simulink model "warplab_mimo_4x4"  (Simulink 6.6)
settings: Solver=ode45  StartTime=0.0  StopTime=50000  RelTol=1e-3
undefined symbols (not defined in the file): gcbh, xlBlockLoadCallback, xlGetSimulinkPeriod
libraries: xbsIndex_r4 x305, WARP_Blockset x16
(part 1 of 4)
settings Model: Creator=mduarte  LastModifiedBy=mduarte

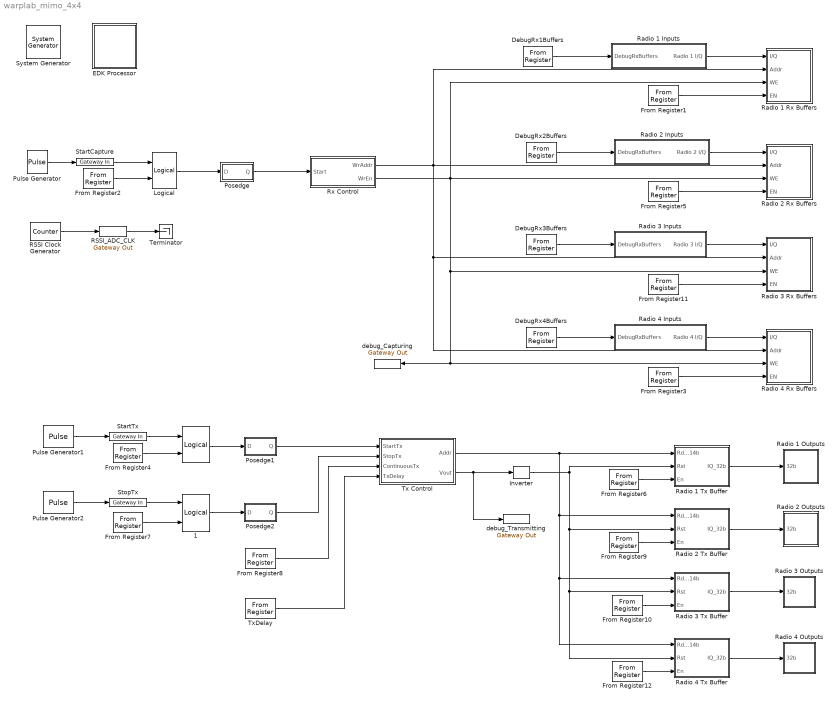
== system warplab_mimo_4x4 ==
  " " : xbsIndex_r4/Logical  logical_function=OR  inputs=2  en=off  latency=0  precision=Full  arith_type=Unsigned  n_bits=16  bin_pt=0  align_bp=on  dbl_ovrd=off  block_type=logical
      settings: block_version=9.1.01
  " 1" : xbsIndex_r4/Logical  logical_function=OR  inputs=2  en=off  latency=0  precision=Full  arith_type=Unsigned  n_bits=16  bin_pt=0  align_bp=on  dbl_ovrd=off  block_type=logical
      settings: block_version=9.1.01
  " System Generator" : xbsIndex_r4/ System Generator  Tag=genX  SystemSampleTime=-1  xilinxfamily=virtex2p  part=xc2vp70  speed=-6  package=ff1517  synthesis_tool=XST  clock_wrapper=Clock Enables  directory=./netlist  testbench=off  simulink_period=1  sysclk_period=10  dcm_input_clock_period=100  incr_netlist=off  trim_vbits=Everywhere in SubSystem  dbl_ovrd=According to Block Masks  core_generation=According to Block Masks  run_coregen=off  deprecated_control=off  eval_field=0  block_type=sysgen
      settings: block_version=10.1.3
  DebugRx1Buffers : xbsIndex_r4/From Register  shared_memory_name='DebugRx1Buffers'  init=0  period=1  ownership=Locally owned and initialized  arith_type=Unsigned  n_bits=1  bin_pt=0  dbl_ovrd=off  block_type=fromreg
      settings: AttributesFormatString=<< %<shared_memory_name> >>  infoedit="Register block that reads data to a shared memory register.  Delay of one sample period."  block_version=10.1.2
  DebugRx2Buffers : xbsIndex_r4/From Register  shared_memory_name='DebugRx2Buffers'  init=0  period=1  ownership=Locally owned and initialized  arith_type=Unsigned  n_bits=1  bin_pt=0  dbl_ovrd=off  block_type=fromreg
      settings: AttributesFormatString=<< %<shared_memory_name> >>  infoedit="Register block that reads data to a shared memory register.  Delay of one sample period."  block_version=10.1.2
  DebugRx3Buffers : xbsIndex_r4/From Register  shared_memory_name='DebugRx3Buffers'  init=0  period=1  ownership=Locally owned and initialized  arith_type=Unsigned  n_bits=1  bin_pt=0  dbl_ovrd=off  block_type=fromreg
      settings: AttributesFormatString=<< %<shared_memory_name> >>  infoedit="Register block that reads data to a shared memory register.  Delay of one sample period."  block_version=10.1.2
  DebugRx4Buffers : xbsIndex_r4/From Register  shared_memory_name='DebugRx4Buffers'  init=0  period=1  ownership=Locally owned and initialized  arith_type=Unsigned  n_bits=1  bin_pt=0  dbl_ovrd=off  block_type=fromreg
      settings: AttributesFormatString=<< %<shared_memory_name> >>  infoedit="Register block that reads data to a shared memory register.  Delay of one sample period."  block_version=10.1.2
  EDK Processor : Subsystem  LoadFcn=xlBlockLoadCallback(gcbh);  mask(Xilinx EDK Processor Block){mode=EDK pcore generation, xmp=, MemVisToProc=<qt bgcolor="#FFFFFF"><div><img src="C:\Xilinx\10.1\DSP_Tools\sysgen\data\images\registerplus.gif"> &lt;&lt;CaptureDone&gt;&gt;<br></div><div><img src="C:\Xilinx\10.1\DSP_Tools\sysgen\data\images\registerplus.gif"> &lt;&lt;DebugRx1Buffers&gt;&gt;<br></div><div><img src="C:\Xilinx\10.1\DSP_Tools\sysgen\data\images\registerplus.gif"> &lt;&lt;DebugRx2Buffers&gt;&gt;<br></div><div><img src="C:\Xilinx\10.1\DSP_Tools\sysgen\data\images\registerplus.gif"> &lt;&lt;DebugRx3Buffers&gt;&gt;<br></div><div><img src="C:\Xilinx\10.1\DSP_Tools\sysgen\data\images\registerplus.gif"> &lt;&lt;DebugRx4Buffers&gt;&gt;<br></div><div><img src="C:\Xilinx\10.1\DSP_Tools\sysgen\data\images\registerplus.gif"> &lt;&lt;RADIO1RXBUFF_RXEN&gt;&gt;<br></div><div><img src="C:\Xilinx\10.1\DSP_Tools\sysgen\data\images\registerplus.gif"> &lt;&lt;RADIO1TXBUFF_TXEN&gt;&gt;<br></div><div><img src="C:\Xilinx\10.1\DSP_Tools\sysgen\data\images\registerplus.gif"> &lt;&lt;RADIO2RXBUFF_RXEN&gt;&gt;<br></div><div><img src="C:\Xilinx\10.1\DSP_Tools\sysgen\data\images\registerplus.gif"> &lt;&lt;RADIO2TXBUFF_TXEN&gt;&gt;<br></div><div><img src="C:\Xilinx\10.1\DSP_Tools\sysgen\data\images\registerplus.gif"> &lt;&lt;RADIO3RXBUFF_RXEN&gt;&gt;<br></div><div><img src="C:\Xilinx\10.1\DSP_Tools\sysgen\data\images\registerplus.gif"> &lt;&lt;RADIO3TXBUFF_TXEN&gt;&gt;<br></div><div><img src="C:\Xilinx\10.1\DSP_Tools\sysgen\data\images\registerplus.gif"> &lt;&lt;RADIO4RXBUFF_RXEN&gt;&gt;<br></div><div><img src="C:\Xilinx\10.1\DSP_Tools\sysgen\data\images\registerplus.gif"> &lt;&lt;RADIO4TXBUFF_TXEN&gt;&gt;<br></div><div><img src="C:\Xilinx\10.1\DSP_Tools\sysgen\data\images\registerplus.gif"> &lt;&lt;StartCapture&gt;&gt;<br></div><div><img src="C:\Xilinx\10.1\DSP_Tools\sysgen\data\images\registerplus.gif"> &lt;&lt;StartTx&gt;&gt;<br></div><div><img src="C:\Xilinx\10.1\DSP_Tools\sysgen\data\images\registerplus.gif"> &lt;&lt;StopTx&gt;&gt;<br></div><div><img src="C:\Xilinx\10.1\DSP_Tools\sysgen\data\images\registerplus.gif"> &lt;&lt;TransMode&gt;&gt;<br></div><div><img src="C:\Xilinx\10.1\DSP_Tools\sysgen\data\images\registerplus.gif"> &lt;&lt;TxDelay&gt;&gt;<br></div><div><img src="C:\Xilinx\10.1\DSP_Tools\sysgen\data\images\registerplus.gif"> &lt;&lt;TxLength&gt;&gt;<br></div><div><img src="C:\Xilinx\10.1\DSP_Tools\sysgen\data\images\memoryplus.gif"> &lt;&lt;RxBuff_Radio1&gt;&gt;<br></div><div><img src="C:\Xilinx\10.1\DSP_Tools\sysgen\data\images\memoryplus.gif"> &lt;&lt;RxBuff_Radio2&gt;&gt;<br></div><div><img src="C:\Xilinx\10.1\DSP_Tools\sysgen\data\images\memoryplus.gif"> &lt;&lt;RxBuff_Radio3&gt;&gt;<br></div><div><img src="C:\Xilinx\10.1\DSP_Tools\sysgen\data\images\memoryplus.gif"> &lt;&lt;RxBuff_Radio4&gt;&gt;<br></div><div><img src="C:\Xilinx\10.1\DSP_Tools\sysgen\data\images\memoryplus.gif"> &lt;&lt;TxBuff_Radio1&gt;&gt;<br></div><div><img src="C:\Xilinx\10.1\DSP_Tools\sysgen\data\images\memoryplus.gif"> &lt;&lt;TxBuff_Radio2&gt;&gt;<br></div><div><img src="C:\Xilinx\10.1\DSP_Tools\sysgen\data\images\memoryplus.gif"> &lt;&lt;TxBuff_Radio3&gt;&gt;<br></div><div><img src="C:\Xilinx\10.1\DSP_Tools\sysgen\data\images\memoryplus.gif"> &lt;&lt;TxBuff_Radio4&gt;&gt;<br></div></qt>, AvailableMemories=<empty>, portInterfaceTable={'exposed'=>[],'portdir'=>[],'portname'=>[],'shortname'=>[]}, bus_type_sgadvanced=, bus_type=PLB, baseaddr=0x80000000, baseaddr_lock_sgadvanced=, baseaddr_lock=off, dual_clock_sgadvanced=, dual_clock=on, reg_readback_sgadvanced=, reg_readback=on, ucf_file=, inheritDeviceType_sgadvanced=, inheritDeviceType=off, clock_name=plb, internalPortList={}, resetPolarity=0, memxtable=|, procinfo={'xmliface'=>'Xilinx//microblaze//iface.xml'}, memmapdirty=off, blockname=, xpsintstyle=default, has_advanced_control=0, sggui_pos=20,20,383,441, block_type=edkprocessor, block_version=2.5, sg_icon_stat=62,64,-1,-1,white,blue,0,07734,right, sg_mask_display=|, sg_list_contents={'table'=>{'AvailableMemories'=>'popup(<empty>)','userSelections'=>{'AvailableMemories'=>'<empty>'}}}, sg_blockgui_xml=}
      mask memxtable=|
      | {'mlist'=>['warplab_mimo_4x4/Rx Control/To Register','warplab_mimo_4x4/DebugRx1Buffers','warplab_mimo_4x4/DebugRx2Buffers','warplab_mimo_4x4/DebugRx3Buffers','warplab_mimo_4x4/DebugRx4Buffers','warplab_mimo_4x4/From Register1','warplab_mimo_4x4/From Register6','warplab_mimo_4x4/From Register5','warplab_mimo_4x4/From Register9','warplab_mimo_4x4/From Register11','warplab_mimo_4x4/From Register10','warplab_mimo_4x4/From Register3','warplab_mimo_4x4/From Register12','warplab_mimo_4x4/From Register2','warplab_mimo_4x4/From Register4','warplab_mimo_4x4/From Register7','warplab_mimo_4x4/From Register8','warplab_mimo_4x4/TxDelay','warplab_mimo_4x4/Tx Control/From Register4','warplab_mimo_4x4/Radio 1
      | Rx Buffers/Radio 1 I//Q
      | Buffer/Shared Memory','warplab_mimo_4x4/Radio 2
      | Rx Buffers/Radio 2 I//Q
      | Buffer/Shared Memory','warplab_mimo_4x4/Radio 3
      | Rx Buffers/Radio 3 I//Q
      | Buffer/Shared Memory','warplab_mimo_4x4/Radio 4
      | Rx Buffers/Radio 4 I//Q
      | Buffer/Shared Memory','warplab_mimo_4x4/Radio 1
      | Tx Buffer/Shared Memory','warplab_mimo_4x4/Radio 2
      | Tx Buffer/Shared Memory','warplab_mimo_4x4/Radio 3
      | Tx Buffer/Shared Memory','warplab_mimo_4x4/Radio 4
      | Tx Buffer/Shared Memory'],'mlname'=>['\'CaptureDone\'','\'DebugRx1Buffers\'','\'DebugRx2Buffers\'','\'DebugRx3Buffers\'','\'DebugRx4Buffers\'','\'RADIO1RXBUFF_RXEN\'','\'RADIO1TXBUFF_TXEN\'','\'RADIO2RXBUFF_RXEN\'','\'RADIO2TXBUFF_TXEN\'','\'RADIO3RXBUFF_RXEN\'','\'RADIO3TXBUFF_TXEN\'','\'RADIO4RXBUFF_RXEN\'','\'RADIO4TXBUFF_TXEN\'','\'StartCapture\'','\'StartTx\'','\'StopTx\'','\'TransMode\'','\'TxDelay\'','\'TxLength\'','\'RxBuff_Radio1\'','\'RxBuff_Radio2\'','\'RxBuff_Radio3\'','\'RxBuff_Radio4\'','\'TxBuff_Radio1\'','\'TxBuff_Radio2\'','\'TxBuff_Radio3\'','\'TxBuff_Radio4\''],'mlstate'=>[0.00000000000000000,0.00000000000000000,0.00000000000000000,0.00000000000000000,0.00000000000000000,0.00000000000000000,0.00000000000000000,0.00000000000000000,0.00000000000000000,0.00000000000000000,0.00000000000000000,0.00000000000000000,0.00000000000000000,0.00000000000000000,0.00000000000000000,0.00000000000000000,0.00000000000000000,0.00000000000000000,0.00000000000000000,0.00000000000000000,0.00000000000000000,0.00000000000000000,0.00000000000000000,0.00000000000000000,0.00000000000000000,0.00000000000000000,0.00000000000000000]}
      mask sg_mask_display=|
      | fprintf('','COMMENT: begin icon graphics');
      | patch([0 62 62 0 ],[0 0 64 64 ],[0.77 0.82 0.91]);
      | patch([14 4 19 4 14 30 34 38 56 42 29 19 33 19 29 42 56 38 34 30 14 ],[8 18 33 48 58 58 54 58 58 44 57 47 33 19 9 22 8 8 12 8 8 ],[0.98 0.96 0.92]);
      | plot([0 62 62 0 0 ],[0 0 64 64 0 ]);
      | fprintf('','COMMENT: end icon graphics');
      | fprintf('','COMMENT: begin icon text');
      | fprintf('','COMMENT: end icon text');
      mask prompts: mode "Configure Processor for"; xmp "EDK Project"; MemVisToProc ""; AvailableMemories "Available Memories"; portInterfaceTable ""; bus_type_sgadvanced ""; bus_type "Bus Type"; baseaddr "Base Address"; baseaddr_lock_sgadvanced ""; baseaddr_lock "Lock"; dual_clock_sgadvanced ""; dual_clock "Dual Clocks"; reg_readback_sgadvanced ""; reg_readback "Register Read-Back"; ucf_file "Constraint file"; inheritDeviceType_sgadvanced ""; inheritDeviceType "Inherit Device Type"; clock_name ""; internalPortList ""; resetPolarity ""; memxtable ""; procinfo ""; memmapdirty ""; blockname ""; xpsintstyle ""; has_advanced_control ""; sggui_pos ""; block_type ""; block_version ""; sg_icon_stat ""; sg_mask_display ""; sg_list_contents ""; sg_blockgui_xml ""
      mask help: Xilinx EDK Processor
      mask init:
      | try
      |   tmp_gcb = gcb;
      |   tmp_gcbh = gcbh;
      |   if (strcmp('SysGenIndex',get_param(bdroot(tmp_gcbh),'tag')) && ~isempty(regexp(bdroot(tmp_gcb), '^xbs', 'once')))
      |     return;
      |   end;
      |   xlMungeMaskParams;
      | 
      | block_type='edkprocessor';
      |   serialized_declarations = '{,''block_type''=>''String''}';
      |   xledkprocessor_init();
      |   ptable_ = xlblockprep(get_param(tmp_gcb, 'MaskWSVariables'));
      | catch
      |   global dbgsysgen;
      |   if(~isempty(dbgsysgen) && dbgsysgen)
      |     e = regexprep(lasterr, '\n', '\nError: ');
      |     disp(['Error: While running MaskInit code on block ' tmp_gcb ': ' e]);
      |     error(e);
      |   end
      | end
      settings: CopyFcn=xlProcBlockCopyCallback(gcbh);xlBlockMoveCallback(gcbh);  DeleteFcn=xlDestroyGui(gcbh);  ModelCloseFcn=xlDestroyGui(gcbh);  PreSaveFcn=xlBlockPreSaveCallback(gcbh);  PostSaveFcn=xlBlockPostSaveCallback(gcbh);  DestroyFcn=xlDestroyGui(gcbh);  OpenFcn=bh=gcbh;xlProcBlockCallbacks('populatesharedmemorylistbox',bh);xlOpenGui(bh, 'edkprocessor_gui.xml', @xlProcBlockEnablement, @xlProcBlockAction)  CloseFcn=xlDestroyGui(gcbh);  MoveFcn=xlBlockMoveCallback(gcbh);
      mask Help: eval('');xlDoc('-book','sysgen','-topic','EDK_Processor');
      mask StyleString: popup(EDK pcore generation|HDL netlisting),edit,edit,popup(<empty>),edit,edit,popup(PLB|FSL),edit,edit,checkbox,edit,checkbox,edit,checkbox,edit,edit,checkbox,edit,edit,edit,edit,edit,edit,edit,edit,edit,edit,edit,edit,edit,edit,edit,edit
      mask Display:
      | fprintf('','COMMENT: begin icon graphics');
      | patch([0 62 62 0 ],[0 0 64 64 ],[0.77 0.82 0.91]);
      | patch([14 4 19 4 14 30 34 38 56 42 29 19 33 19 29 42 56 38 34 30 14 ],[8 18 33 48 58 58 54 58 58 44 57 47 33 19 9 22 8 8 12 8 8 ],[0.98 0.96 0.92]);
      | plot([0 62 62 0 0 ],[0 0 64 64 0 ]);
      | fprintf('','COMMENT: end icon graphics');
      | fprintf('','COMMENT: begin icon text');
      | disp('');
      | 
      | fprintf('','COMMENT: end icon text');
  From Register1 : xbsIndex_r4/From Register  shared_memory_name='RADIO1RXBUFF_RXEN'  init=0  period=1  ownership=Locally owned and initialized  arith_type=Unsigned  n_bits=1  bin_pt=0  dbl_ovrd=off  block_type=fromreg
      settings: AttributesFormatString=RADIO1RXBUFF_RXEN\n<< %<shared_memory_name> >>  infoedit="Register block that reads data to a shared memory register.  Delay of one sample period."  block_version=8.2
  From Register10 : xbsIndex_r4/From Register  shared_memory_name='RADIO3TXBUFF_TXEN'  init=0  period=1  ownership=Locally owned and initialized  arith_type=Unsigned  n_bits=1  bin_pt=0  dbl_ovrd=off  block_type=fromreg
      settings: AttributesFormatString=RADIO3TXBUFF_TXEN\n<< %<shared_memory_name> >>  infoedit="Register block that reads data to a shared memory register.  Delay of one sample period."  block_version=8.2
  From Register11 : xbsIndex_r4/From Register  shared_memory_name='RADIO3RXBUFF_RXEN'  init=0  period=1  ownership=Locally owned and initialized  arith_type=Unsigned  n_bits=1  bin_pt=0  dbl_ovrd=off  block_type=fromreg
      settings: AttributesFormatString=RADIO3RXBUFF_RXEN\n<< %<shared_memory_name> >>  infoedit="Register block that reads data to a shared memory register.  Delay of one sample period."  block_version=8.2
  From Register12 : xbsIndex_r4/From Register  shared_memory_name='RADIO4TXBUFF_TXEN'  init=0  period=1  ownership=Locally owned and initialized  arith_type=Unsigned  n_bits=1  bin_pt=0  dbl_ovrd=off  block_type=fromreg
      settings: AttributesFormatString=RADIO4TXBUFF_TXEN\n<< %<shared_memory_name> >>  infoedit="Register block that reads data to a shared memory register.  Delay of one sample period."  block_version=8.2
  From Register2 : xbsIndex_r4/From Register  shared_memory_name='StartCapture'  init=0  period=1  ownership=Locally owned and initialized  arith_type=Unsigned  n_bits=1  bin_pt=0  dbl_ovrd=off  block_type=fromreg
      settings: AttributesFormatString=StartCapture\n<< %<shared_memory_name> >>  infoedit="Register block that reads data to a shared memory register.  Delay of one sample period."  block_version=8.2
  From Register3 : xbsIndex_r4/From Register  shared_memory_name='RADIO4RXBUFF_RXEN'  init=0  period=1  ownership=Locally owned and initialized  arith_type=Unsigned  n_bits=1  bin_pt=0  dbl_ovrd=off  block_type=fromreg
      settings: AttributesFormatString=RADIO4RXBUFF_RXEN\n<< %<shared_memory_name> >>  infoedit="Register block that reads data to a shared memory register.  Delay of one sample period."  block_version=8.2
  From Register4 : xbsIndex_r4/From Register  shared_memory_name='StartTx'  init=0  period=1  ownership=Locally owned and initialized  arith_type=Unsigned  n_bits=1  bin_pt=0  dbl_ovrd=off  block_type=fromreg
      settings: AttributesFormatString=StartTx\n<< %<shared_memory_name> >>  infoedit="Register block that reads data to a shared memory register.  Delay of one sample period."  block_version=8.2
  From Register5 : xbsIndex_r4/From Register  shared_memory_name='RADIO2RXBUFF_RXEN'  init=0  period=1  ownership=Locally owned and initialized  arith_type=Unsigned  n_bits=1  bin_pt=0  dbl_ovrd=off  block_type=fromreg
      settings: AttributesFormatString=RADIO2RXBUFF_RXEN\n<< %<shared_memory_name> >>  infoedit="Register block that reads data to a shared memory register.  Delay of one sample period."  block_version=8.2
  From Register6 : xbsIndex_r4/From Register  shared_memory_name='RADIO1TXBUFF_TXEN'  init=0  period=1  ownership=Locally owned and initialized  arith_type=Unsigned  n_bits=1  bin_pt=0  dbl_ovrd=off  block_type=fromreg
      settings: AttributesFormatString=RADIO1TXBUFF_TXEN\n<< %<shared_memory_name> >>  infoedit="Register block that reads data to a shared memory register.  Delay of one sample period."  block_version=8.2
  From Register7 : xbsIndex_r4/From Register  shared_memory_name='StopTx'  init=0  period=1  ownership=Locally owned and initialized  arith_type=Unsigned  n_bits=1  bin_pt=0  dbl_ovrd=off  block_type=fromreg
      settings: AttributesFormatString=StopTx\n<< %<shared_memory_name> >>  infoedit="Register block that reads data to a shared memory register.  Delay of one sample period."  block_version=8.2
  From Register8 : xbsIndex_r4/From Register  shared_memory_name='TransMode'  init=0  period=1  ownership=Locally owned and initialized  arith_type=Unsigned  n_bits=1  bin_pt=0  dbl_ovrd=off  block_type=fromreg
      settings: AttributesFormatString=TransMode\n<< %<shared_memory_name> >>  infoedit="Register block that reads data to a shared memory register.  Delay of one sample period."  block_version=8.2
  From Register9 : xbsIndex_r4/From Register  shared_memory_name='RADIO2TXBUFF_TXEN'  init=0  period=1  ownership=Locally owned and initialized  arith_type=Unsigned  n_bits=1  bin_pt=0  dbl_ovrd=off  block_type=fromreg
      settings: AttributesFormatString=RADIO2TXBUFF_TXEN\n<< %<shared_memory_name> >>  infoedit="Register block that reads data to a shared memory register.  Delay of one sample period."  block_version=8.2
  Inverter : xbsIndex_r4/Inverter  en=off  latency=0  dbl_ovrd=off  block_type=inv
      settings: block_version=8.2
  Logical : xbsIndex_r4/Logical  logical_function=OR  inputs=2  en=off  latency=0  precision=Full  arith_type=Unsigned  n_bits=16  bin_pt=0  align_bp=on  dbl_ovrd=off  block_type=logical
      settings: block_version=8.2
  Posedge : Subsystem
  Posedge1 : Subsystem
  Posedge2 : Subsystem
  Pulse Generator : DiscretePulseGenerator  Period=1000000  PulseWidth=50  PhaseDelay=2
  Pulse Generator1 : DiscretePulseGenerator  Period=10 * 2^14  PulseWidth=50  PhaseDelay=2
  Pulse Generator2 : DiscretePulseGenerator  Period=10 * 2^14  PulseWidth=50  PhaseDelay=2.5 * 2^14
  RSSI Clock Generator : xbsIndex_r4/Counter  cnt_type=Free Running  cnt_to=Inf  operation=Up  start_count=0  cnt_by_val=1  arith_type=Unsigned  n_bits=1  bin_pt=0  load_pin=off  rst=off  en=off  explicit_period=on  period=2  dbl_ovrd=off  use_behavioral_HDL=off  use_rpm=off  implementation=Fabric  block_type=counter
      settings: block_version=VER_STRING_GOES_HERE
  RSSI_ADC_CLK : xbsIndex_r4/Gateway Out  hdl_port=on  timing_constraint=None  locs_specified=off  LOCs={}  block_type=gatewayout
      settings: infoedit="Gateway out block.  Converts Xilinx fixed point inputs into ouputs of type Simulink integer, double, or fixed point.<P><P>Hardware notes:  In hardware these blocks become top level output ports or are discarded, depending on how they are configured."  block_version=8.2
  Radio 1 Rx Buffers : Subsystem
  Radio 1 Tx Buffer : Subsystem
  Radio 1 Inputs : Subsystem
  Radio 1 Outputs : Subsystem
  Radio 2 Rx Buffers : Subsystem
  Radio 2 Tx Buffer : Subsystem
  Radio 2 Inputs : Subsystem
  Radio 2 Outputs : Subsystem
  Radio 3 Rx Buffers : Subsystem
  Radio 3 Tx Buffer : Subsystem
  Radio 3 Inputs : Subsystem
  Radio 3 Outputs : Subsystem
  Radio 4 Rx Buffers : Subsystem
  Radio 4 Tx Buffer : Subsystem
  Radio 4 Inputs : Subsystem
  Radio 4 Outputs : Subsystem
  Rx Control : Subsystem
  StartCapture : xbsIndex_r4/Gateway In  arith_type=Unsigned  n_bits=1  bin_pt=0  quantization="Round  (unbiased: +/- Inf)"  overflow=Saturate  period=1  dbl_ovrd=off  timing_constraint=None  locs_specified=off  LOCs={}  block_type=gatewayin
      settings: infoedit="Gateway in block.  Converts inputs of type Simulink integer, double and fixed point to  Xilinx fixed point type.<P><P>Hardware notes:  In hardware these blocks become top level input ports."  block_version=VER_STRING_GOES_HERE
  StartTx : xbsIndex_r4/Gateway In  arith_type=Unsigned  n_bits=1  bin_pt=0  quantization="Round  (unbiased: +/- Inf)"  overflow=Saturate  period=1  dbl_ovrd=off  timing_constraint=None  locs_specified=off  LOCs={}  block_type=gatewayin
      settings: infoedit="Gateway in block.  Converts inputs of type Simulink integer, double and fixed point to  Xilinx fixed point type.<P><P>Hardware notes:  In hardware these blocks become top level input ports."  block_version=VER_STRING_GOES_HERE
  StopTx : xbsIndex_r4/Gateway In  arith_type=Unsigned  n_bits=1  bin_pt=0  quantization="Round  (unbiased: +/- Inf)"  overflow=Saturate  period=1  dbl_ovrd=off  timing_constraint=None  locs_specified=off  LOCs={}  block_type=gatewayin
      settings: infoedit="Gateway in block.  Converts inputs of type Simulink integer, double and fixed point to  Xilinx fixed point type.<P><P>Hardware notes:  In hardware these blocks become top level input ports."  block_version=VER_STRING_GOES_HERE
  Terminator : Terminator
  Tx Control : Subsystem
  TxDelay : xbsIndex_r4/From Register  shared_memory_name='TxDelay'  init=1000  period=1  ownership=Locally owned and initialized  arith_type=Unsigned  n_bits=14  bin_pt=0  dbl_ovrd=off  block_type=fromreg
      settings: AttributesFormatString=<< %<shared_memory_name> >>  infoedit="Register block that reads data to a shared memory register.  Delay of one sample period."  block_version=10.1.2
  debug_Capturing : xbsIndex_r4/Gateway Out  Orientation=left  hdl_port=on  timing_constraint=None  locs_specified=off  LOCs={}  block_type=gatewayout
      settings: infoedit="Gateway out block.  Converts Xilinx fixed point inputs into ouputs of type Simulink integer, double, or fixed point.<P><P>Hardware notes:  In hardware these blocks become top level output ports or are discarded, depending on how they are configured."  block_version=8.2
  debug_Transmitting : xbsIndex_r4/Gateway Out  hdl_port=on  timing_constraint=None  locs_specified=off  LOCs={}  block_type=gatewayout
      settings: infoedit="Gateway out block.  Converts Xilinx fixed point inputs into ouputs of type Simulink integer, double, or fixed point.<P><P>Hardware notes:  In hardware these blocks become top level output ports or are discarded, depending on how they are configured."  block_version=8.2
  wires:
  Pulse Generator/1 -> StartCapture/1
  From Register2/1 -> Logical/2
  Logical/1 -> Posedge/1(D)
  StartCapture/1 -> Logical/1
  RSSI Clock Generator/1 -> RSSI_ADC_CLK/1
  Radio 3 Inputs/1(Radio 3 I/Q) -> Radio 3 Rx Buffers/1(I/Q)
  From Register11/1 -> Radio 3 Rx Buffers/4(EN)
  Radio 2 Inputs/1(Radio 2 I/Q) -> Radio 2 Rx Buffers/1(I/Q)
  From Register5/1 -> Radio 2 Rx Buffers/4(EN)
  RSSI_ADC_CLK/1 -> Terminator/1
  Posedge/1(Q) -> Rx Control/1(Start)
  DebugRx2Buffers/1 -> Radio 2 Inputs/1(DebugRxBuffers)
  DebugRx3Buffers/1 -> Radio 3 Inputs/1(DebugRxBuffers)
  Radio 1 Inputs/1(Radio 1 I/Q) -> Radio 1 Rx Buffers/1(I/Q)
  From Register1/1 -> Radio 1 Rx Buffers/4(EN)
  DebugRx1Buffers/1 -> Radio 1 Inputs/1(DebugRxBuffers)
  Radio 4 Inputs/1(Radio 4 I/Q) -> Radio 4 Rx Buffers/1(I/Q)
  From Register3/1 -> Radio 4 Rx Buffers/4(EN)
  DebugRx4Buffers/1 -> Radio 4 Inputs/1(DebugRxBuffers)
  Rx Control/1(WrAddr) -> Radio 2 Rx Buffers/2(Addr), Radio 1 Rx Buffers/2(Addr), Radio 3 Rx Buffers/2(Addr), Radio 4 Rx Buffers/2(Addr)
  Rx Control/2(WrEn) -> Radio 2 Rx Buffers/3(WE), Radio 3 Rx Buffers/3(WE), Radio 4 Rx Buffers/3(WE), debug_Capturing/1, Radio 1 Rx Buffers/3(WE)
  Radio 2 Tx Buffer/1(IQ_32b) -> Radio 2 Outputs/1(32b)
  Posedge1/1(Q) -> Tx Control/1(StartTx)
  From Register4/1 -> " "/2
  From Register7/1 -> " 1"/2
  From Register8/1 -> Tx Control/3(ContinuousTx)
  Posedge2/1(Q) -> Tx Control/2(StopTx)
  " 1"/1 -> Posedge2/1(D)
  StopTx/1 -> " 1"/1
  Pulse Generator2/1 -> StopTx/1
  " "/1 -> Posedge1/1(D)
  StartTx/1 -> " "/1
  Pulse Generator1/1 -> StartTx/1
  From Register9/1 -> Radio 2 Tx Buffer/3(En)
  TxDelay/1 -> Tx Control/4(TxDelay)
  Tx Control/2(Vout) -> debug_Transmitting/1, Inverter/1
  Radio 3 Tx Buffer/1(IQ_32b) -> Radio 3 Outputs/1(32b)
  From Register10/1 -> Radio 3 Tx Buffer/3(En)
  Radio 1 Tx Buffer/1(IQ_32b) -> Radio 1 Outputs/1(32b)
  From Register6/1 -> Radio 1 Tx Buffer/3(En)
  Radio 4 Tx Buffer/1(IQ_32b) -> Radio 4 Outputs/1(32b)
  From Register12/1 -> Radio 4 Tx Buffer/3(En)
  Tx Control/1(Addr) -> Radio 1 Tx Buffer/1(RdAddr_14b), Radio 2 Tx Buffer/1(RdAddr_14b), Radio 3 Tx Buffer/1(RdAddr_14b), Radio 4 Tx Buffer/1(RdAddr_14b)
  Inverter/1 -> Radio 1 Tx Buffer/2(Rst), Radio 2 Tx Buffer/2(Rst), Radio 3 Tx Buffer/2(Rst), Radio 4 Tx Buffer/2(Rst)
